simulink model "Q3bSL"  (R2020a)
settings: Solver=VariableStepAuto  StartTime=0.0  StopTime=10.0  RelTol=1e-3
InitFcn:
  | cl = 0.6742
  | cd = 0.02
  | gamma_eq = 0.0279
  | V_eq1000 = 38.6349
  | g = 0.81
  | m = 454
  | S = 7.43
libraries: aerolibatmos2 x1
settings Model: Creator=Ali  LastModifiedBy=Ali

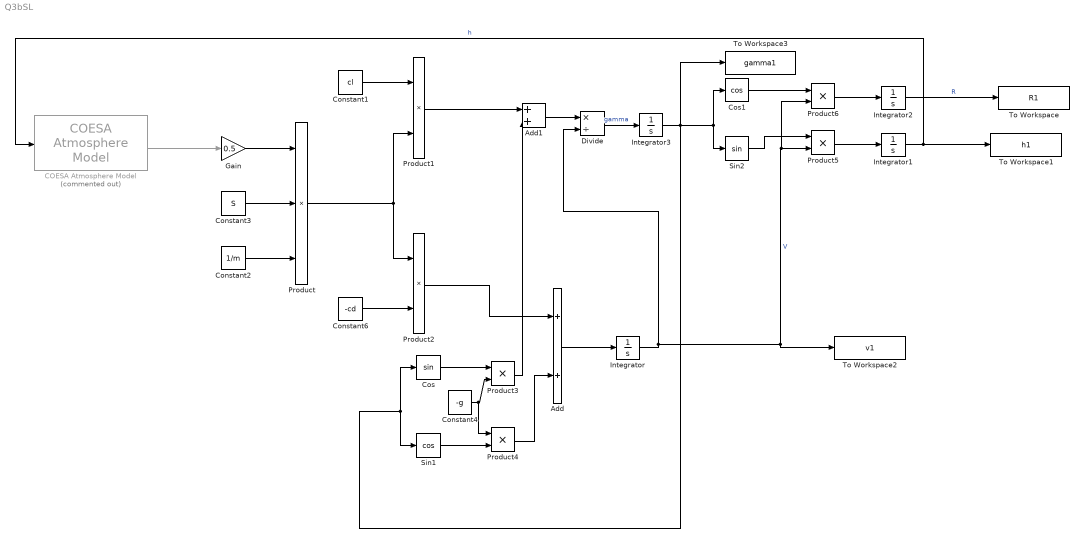
== system Q3bSL ==
  Add : Sum
  Add1 : Sum
  COESA Atmosphere Model : aerolibatmos2/COESA Atmosphere Model  Commented=on  units=Metric (MKS)  spec=1976 COESA-extended U.S. Standard Atmosphere  model=Profile  profile_var=High temperature  profile_percent=1%  profile_alt=5 km (16404 ft)  envelope_var=High temperature  envelope_percent=1%  action=Warning
  Constant1 : Constant  Value=cl
  Constant2 : Constant  Value=1/m
  Constant3 : Constant  Value=S
  Constant4 : Constant  Value=-g
  Constant6 : Constant  Value=-cd
  Cos : Trigonometry
  Cos1 : Trigonometry  Operator=cos
  Divide : Product  Inputs=*/
  Gain : Gain  Gain=0.5
  Integrator : Integrator  InitialCondition=V_eq1000*0.3048
  Integrator1 : Integrator  InitialCondition=1000*0.3048
  Integrator2 : Integrator
  Integrator3 : Integrator
  Product : Product  Inputs=3
  Product{1..6} (6 alike) : Product
  Sin1 : Trigonometry  Operator=cos
  Sin2 : Trigonometry
  To Workspace : ToWorkspace  VariableName=R1  SaveFormat=Timeseries  SampleTime=-1
  To Workspace1 : ToWorkspace  VariableName=h1  SaveFormat=Timeseries  SampleTime=-1
  To Workspace2 : ToWorkspace  VariableName=v1  SaveFormat=Timeseries  SampleTime=-1
  To Workspace3 : ToWorkspace  VariableName=gamma1  SaveFormat=Timeseries  SampleTime=-1
  wires:
  COESA Atmosphere Model/3 -> Gain/1
  Gain/1 -> Product/1
  Constant3/1 -> Product/2
  Constant2/1 -> Product/3
  Constant1/1 -> Product1/1
  Product/1 -> Product2/1, Product1/2
  Constant6/1 -> Product2/2
  Constant4/1 -> Product4/1, Product3/2
  Cos/1 -> Product3/1
  Sin1/1 -> Product4/2
  Product2/1 -> Add/1
  Add/1 -> Integrator/1
  Integrator/1 -> Product6/2, Product5/2, To Workspace2/1, Divide/2  "V"
  Product1/1 -> Add1/1
  Product4/1 -> Add/2
  Product3/1 -> Add1/2
  Add1/1 -> Divide/1
  Divide/1 -> Integrator3/1  "gamma"
  Sin2/1 -> Product5/1
  Product5/1 -> Integrator1/1
  Cos1/1 -> Product6/1
  Product6/1 -> Integrator2/1
  Integrator2/1 -> To Workspace/1  "R"
  Integrator1/1 -> To Workspace1/1, COESA Atmosphere Model/1  "h"
  Integrator3/1 -> To Workspace3/1, Cos/1, Sin1/1, Cos1/1, Sin2/1
